simulink library "makeOcB_cl"  (R2018b)
settings: Solver=VariableStepAuto  StartTime=0.0  StopTime=10.0  RelTol=1e-3
libraries: rotationAboutX x1, rotationAboutY x1, rotationAboutZ x1
settings Model: Creator=Ayaz  LastModifiedBy=Ayaz
settings DataIOCC: ReturnWorkspaceOutputs=on

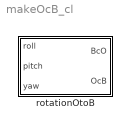
== system makeOcB_cl ==
  rotationOtoB : Subsystem

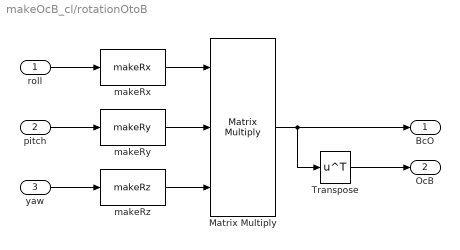
== system makeOcB_cl/rotationOtoB ==
  roll : Inport
  pitch : Inport  Port=2
  yaw : Inport  Port=3
  Matrix Multiply : Product  Inputs=3  Multiplication=Matrix(*)
  Transpose : Math  Operator=transpose  SaturateOnIntegerOverflow=on
  makeRx : rotationAboutX/makeRx  SystemSampleTime=-1  Latency=0  AutoFrameSizeCalculation=off
  makeRy : rotationAboutY/makeRy  SystemSampleTime=-1  Latency=0  AutoFrameSizeCalculation=off
  makeRz : rotationAboutZ/makeRz  SystemSampleTime=-1  Latency=0  AutoFrameSizeCalculation=off
  BcO : Outport
  OcB : Outport  Port=2
  wires:
  yaw/1 -> makeRz/1
  roll/1 -> makeRx/1
  pitch/1 -> makeRy/1
  makeRx/1 -> Matrix Multiply/1
  makeRy/1 -> Matrix Multiply/2
  makeRz/1 -> Matrix Multiply/3
  Matrix Multiply/1 -> Transpose/1, BcO/1
  Transpose/1 -> OcB/1
